simulink model "SimulArm_Interpolate"  (R2025b)
settings: Solver=VariableStepAuto  StartTime=0.0  StopTime=35  FixedStep=.02  RelTol=1e-3  AbsTol=1e-3  EnableMultiTasking=on
values from neighbouring files (symbols this model uses):
  C = U * V'    [DataCondition.m]
  g = 9.80665    [DataCondition.m]
  N = numel(raw)    [DataCondition.m]
  roll_offset = 0    [DataCondition.m]
  rot_x_bicep = rot_bicep(:,1)    [DataCondition.m]
  rot_y_bicep = - rot_bicep(:,2)    [DataCondition.m]
  rot_y_wrist = - (rot_wrist(:,2) - rot_bicep(:,2))    [DataCondition.m]
  rot_z_bicep = rot_bicep(:,3)    [DataCondition.m]
  rot_z_wrist = (rot_wrist(:,3) - rot_bicep(:,3))    [DataCondition.m]
  time = time - time(1)    [DataCondition.m]
undefined symbols (not defined in the file or in its folder): X, Y, Z
libraries: sm_lib x45, nesl_utility x24, aerolibconvert2 x10, simulink x1
(part 1 of 3)
settings Model: Creator=ricky  LastModifiedBy=ricky
settings SolverCC: AutoScaleAbsTol=off  AlgebraicLoopSolver=TrustRegion  MaxZcPerStep=1.0
settings DataIOCC: LimitDataPoints=on  MaxDataPoints=10000
settings OptimizationCC: ReuseModelBlockBuffer=off  LifeSpan=inf
settings DebuggingCC: UnconnectedInputMsg=warning  UnconnectedOutputMsg=warning  UnconnectedLineMsg=warning  AllowSymbolicDim=off  SubsystemReferenceDiagnosticForUnitTest=warning  SFUnexpectedBacktrackingDiag=warning  SFNoUnconditionalDefaultTransitionDiag=warning  SFExecutionAtInitializationDiag=none  ArithmeticOperatorsInVariantConditions=warning
settings ModelReferenceCC: EnableRefExpFcnMdlSchedulingChecks=on
settings SFSimCC: SimUseLocalCustomCode=off  CustomCodeUndefinedFunction=UseInterfaceOnly
settings RTWCC: RTWUseLocalCustomCode=off  GPUComputeCapability=3.5  DLArmComputeVersion=19.05
settings CodeAppCC: StateflowObjectComments=on
settings GRTTargetCC: TargetLangStandard=C89/C90 (ANSI)
settings ConfigComp: CovMetricSettings=dw  CovSaveCumulativeToWorkspaceVar=on  CovSaveSingleToWorkspaceVar=on  CovExternalEMLEnable=off  CovSFcnEnable=off
settings SimscapeCC: SimscapeLogType=all  SimscapeLogSimulationStatistics=on  SimscapeLogDataHistory=10000.0

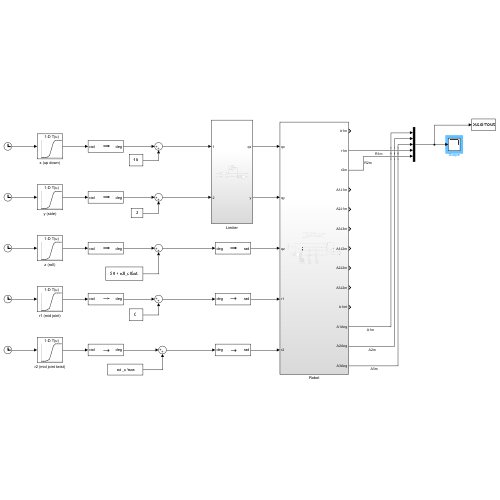
[thumbnail: Simulink's stored preview of the top-level diagram]
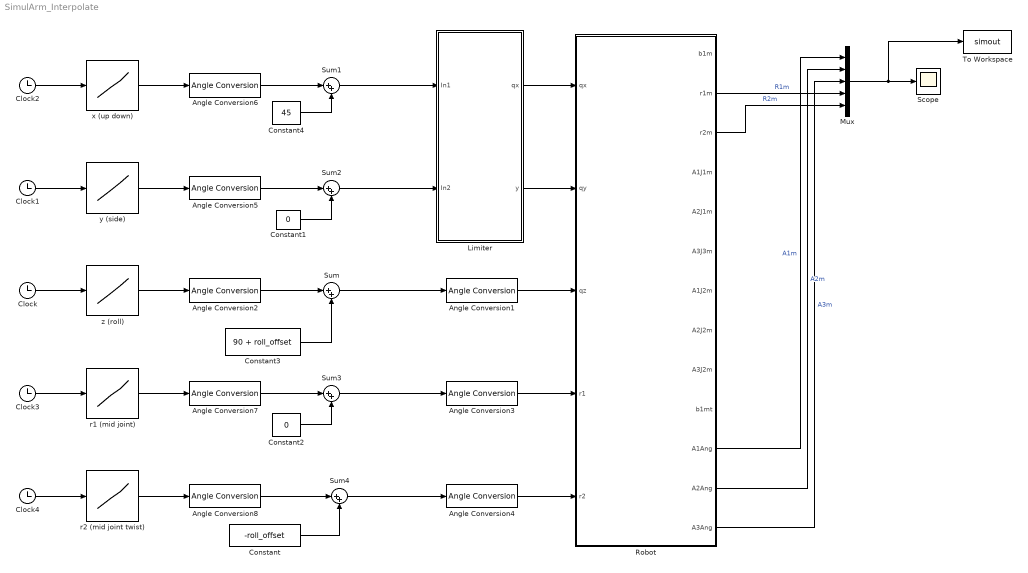
== system SimulArm_Interpolate ==
  Angle Conversion1 : aerolibconvert2/Angle Conversion  IU=deg  OU=rad
  Angle Conversion{2,5..8} (5 alike) : aerolibconvert2/Angle Conversion  IU=rad  OU=deg
  Angle Conversion3 : aerolibconvert2/Angle Conversion  IU=deg  OU=rad
  Angle Conversion4 : aerolibconvert2/Angle Conversion  IU=deg  OU=rad
  Clock{,1..4} (5 alike) : Clock
  Constant : Constant  Value=-roll_offset
  Constant1 : Constant  Value=0
  Constant2 : Constant  Value=0
  Constant3 : Constant  Value=90 + roll_offset
  Constant4 : Constant  Value=45
  Limiter : Subsystem
  Mux : Mux  Inputs=5
  Robot : Subsystem
  Scope : Scope
      settings: Title=Joint Angles vs. Time  ActiveDisplayYMinimum=-4.4475465064355415  ActiveDisplayYMaximum=4.6307923111604765  YLabel=rad
  Sum{,1..4} (5 alike) : Sum  Inputs=|++
  To Workspace : ToWorkspace  VariableName=simout  SaveFormat=Timeseries  SampleTime=-1
  r1 (mid joint) : Lookup_n-D  NumberOfTableDimensions=1  BreakpointsForDimension1=time  Table=rot_y_wrist  ExtrapMethod=Clip  InternalRulePriority=Speed  RndMeth=Simplest
  r2 (mid joint twist) : Lookup_n-D  NumberOfTableDimensions=1  BreakpointsForDimension1=time  Table=rot_z_wrist  ExtrapMethod=Clip  InternalRulePriority=Speed  RndMeth=Simplest
  x (up down) : Lookup_n-D  NumberOfTableDimensions=1  BreakpointsForDimension1=time  Table=rot_x_bicep  ExtrapMethod=Clip  InternalRulePriority=Speed  RndMeth=Simplest
  y (side) : Lookup_n-D  NumberOfTableDimensions=1  BreakpointsForDimension1=time  Table=rot_y_bicep  ExtrapMethod=Clip  InternalRulePriority=Speed  RndMeth=Simplest
  z (roll) : Lookup_n-D  NumberOfTableDimensions=1  BreakpointsForDimension1=time  Table=rot_z_bicep  ExtrapMethod=Clip  InternalRulePriority=Speed  RndMeth=Simplest
  wires:
  Limiter/1(qx) -> Robot/1(qx)
  Angle Conversion1/1 -> Robot/3(qz)
  Sum/1 -> Angle Conversion1/1
  Constant3/1 -> Sum/2
  Constant4/1 -> Sum1/2
  Constant1/1 -> Sum2/2
  Limiter/2(y) -> Robot/2(qy)
  Angle Conversion3/1 -> Robot/4(r1)
  Angle Conversion4/1 -> Robot/5(r2)
  Angle Conversion7/1 -> Sum3/1
  Constant2/1 -> Sum3/2
  Angle Conversion8/1 -> Sum4/1
  Constant/1 -> Sum4/2
  Sum3/1 -> Angle Conversion3/1
  Sum4/1 -> Angle Conversion4/1
  z (roll)/1 -> Angle Conversion2/1
  Angle Conversion6/1 -> Sum1/1
  Angle Conversion5/1 -> Sum2/1
  Angle Conversion2/1 -> Sum/1
  x (up down)/1 -> Angle Conversion6/1
  y (side)/1 -> Angle Conversion5/1
  Clock1/1 -> y (side)/1
  Clock2/1 -> x (up down)/1
  Clock/1 -> z (roll)/1
  Sum1/1 -> Limiter/1(In1)
  Sum2/1 -> Limiter/2(In2)
  r2 (mid joint twist)/1 -> Angle Conversion8/1
  r1 (mid joint)/1 -> Angle Conversion7/1
  Clock4/1 -> r2 (mid joint twist)/1
  Clock3/1 -> r1 (mid joint)/1
  Robot/2(r1m) -> Mux/4  "R1m"
  Robot/3(r2m) -> Mux/5  "R2m"
  Robot/11(A1Ang) -> Mux/1  "A1m"
  Robot/12(A2Ang) -> Mux/2  "A2m"
  Robot/13(A3Ang) -> Mux/3  "A3m"
  Mux/1 -> To Workspace/1, Scope/1

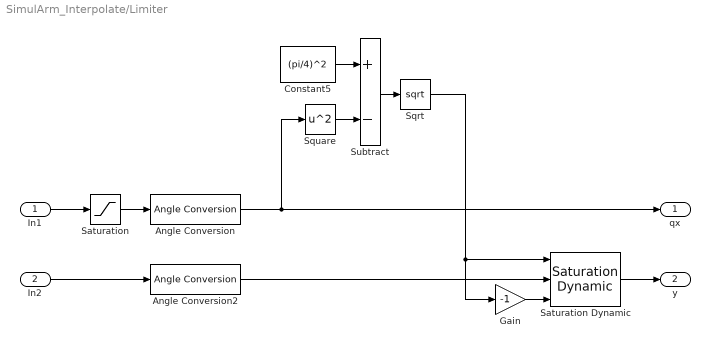
== system SimulArm_Interpolate/Limiter ==
  In1 : Inport
  In2 : Inport  Port=2
  Angle Conversion : aerolibconvert2/Angle Conversion  IU=deg  OU=rad
  Angle Conversion2 : aerolibconvert2/Angle Conversion  IU=deg  OU=rad
  Constant5 : Constant  Value=(pi/4)^2
  Gain : Gain  Gain=-1
  Saturation : Saturate  UpperLimit=45  LowerLimit=-45
  Saturation Dynamic : simulink/Discontinuities/Saturation Dynamic  OutMin=[]  OutMax=[]  OutDataTypeStr=Inherit: Same as second input  OutDataType=fixdt(1, 16)  OutScaling=2^-10  DoSatur=off
  Sqrt : Sqrt
  Square : Math  Operator=square
  Subtract : Sum  Inputs=+-
  qx : Outport
  y : Outport  Port=2
  wires:
  Gain/1 -> Saturation Dynamic/3
  Angle Conversion2/1 -> Saturation Dynamic/2
  Sqrt/1 -> Gain/1, Saturation Dynamic/1
  Subtract/1 -> Sqrt/1
  Constant5/1 -> Subtract/1
  Angle Conversion/1 -> qx/1, Square/1
  Square/1 -> Subtract/2
  In1/1 -> Saturation/1
  Saturation Dynamic/1 -> y/1
  In2/1 -> Angle Conversion2/1
  Saturation/1 -> Angle Conversion/1
